simulink model "Dynamic_motor_model_vs_static_motor_model"  (R2019b)
settings: Solver=VariableStepAuto  StartTime=0.0  StopTime=1  RelTol=1e-3
undefined symbols (not defined in the file): c_e, R_a
settings Model: Creator=Олег  LastModifiedBy=Олег

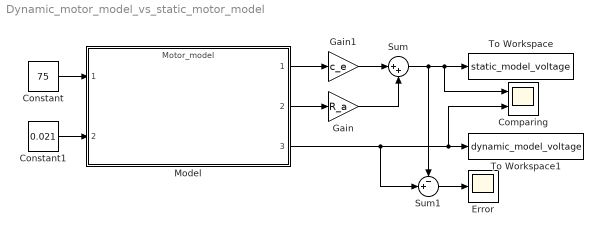
== system Dynamic_motor_model_vs_static_motor_model ==
  Comparing : Scope  NumInputPorts=2
  Constant : Constant  Value=75
  Constant1 : Constant  Value=0.021
  Error : Scope
  Gain : Gain  Gain=R_a
  Gain1 : Gain  Gain=c_e
  Model : ModelReference  ModelNameDialog=Motor_model.slx  SimulationMode=Normal  ModelReferenceVersion=1.137
  Sum : Sum  Inputs=|++
  Sum1 : Sum  Inputs=-+|
  To Workspace : ToWorkspace  VariableName=static_model_voltage  SaveFormat=Timeseries  SampleTime=-1
  To Workspace1 : ToWorkspace  VariableName=dynamic_model_voltage  SaveFormat=Timeseries  SampleTime=-1
  wires:
  Model/2 -> Gain/1
  Model/1 -> Gain1/1
  Gain1/1 -> Sum/1
  Gain/1 -> Sum/2
  Sum/1 -> To Workspace/1, Comparing/1, Sum1/1
  Model/3 -> To Workspace1/1, Comparing/2, Sum1/2
  Sum1/1 -> Error/1
  Constant/1 -> Model/1
  Constant1/1 -> Model/2
